simulink model "IARC_Nonlinear_Sensors"  (R2018a)
settings: Solver=ode1  StartTime=0.0  StopTime=20  FixedStep=T  RelTol=1e-3  EnableMultiTasking=on
undefined symbols (not defined in the file): A_1df, A_2df, alpha3, alpha_rp, alpha_x, alpha_z, an1, an1_v, an2, an3, bn1, bn1_v, bn2, bn3, dc_M_x, delta3, Epsilon3, F, g, Gamma1, Gamma2, Gamma3, Gamma4, gamma4_0, gamma_d_x, gamma_rp_0, gamma_x_0, gamma_z_0, Gammax, I, I_add, I_add_time, Jx, Jy, Jyaw, K, k1, k10, k11, k12, k2, k3, k4, k5, k6, k7, k8, k9, Ky, L, Light, LIMIT_CMD_PITCH, LIMIT_CMD_ROLL, LIMIT_CMD_xy, LIMIT_uCMD_HEIGHT, m, m_add, m_add_time, magnitude, MIL ... (+67)
libraries: simulink x131, simulink_extras x5, UAV_Control x4, aerolibwind2 x1
(part 6 of 6)

== system IARC_Nonlinear_Sensors/ARC Controller/Attitutde Control/pitch control/Adaptation Law_X/IARC, Physical Model Based Parameter Estimation (69)_pitch (theta)/Gamma/InitializationDelay ==
  u : Inport
  Clock : Clock
  Compare To Constant2 : simulink/Logic and Bit Operations/Compare To Constant  relop=>=  const=t0  OutDataTypeStr=boolean
  Data Type Conversion : DataTypeConversion
  Product : Product
  y : Outport
  wires:
  u/1 -> Product/1
  Compare To Constant2/1 -> Data Type Conversion/1
  Clock/1 -> Compare To Constant2/1
  Data Type Conversion/1 -> Product/2
  Product/1 -> y/1

== system IARC_Nonlinear_Sensors/ARC Controller/Attitutde Control/pitch control/Adaptation Law_X/IARC, Physical Model Based Parameter Estimation (69)_pitch (theta)/Gamma/vDv ==
  In1 : Inport
  Product2 : Product  Inputs=3  Multiplication=Matrix(*)
  Transpose2 : Math  Operator=transpose  SaturateOnIntegerOverflow=on
  eigenvector of Gamm_max : Constant  Value=v
  Out1 : Outport
  wires:
  Transpose2/1 -> Product2/1
  In1/1 -> Product2/2
  eigenvector of Gamm_max/1 -> Transpose2/1, Product2/3
  Product2/1 -> Out1/1

== system IARC_Nonlinear_Sensors/ARC Controller/Attitutde Control/roll control/Adaptation Law_Y/IARC, Physical Model Based Parameter Estimation (69)_roll (phi)/Gamma/Gamma_dot ==
  note: D.Gamma=mu1.G-mu2.G.P.P.G
      |
      | Normalized:
      | D.Gamma=alpha.G-(G.P.P.G)/(1+nu.P.GP)
  Phi_f : Inport
  Gamma : Inport  Port=2
  " " : Gain  Gain=mu2
  "  (Normalized)" : Gain  Gain=nu
  Add : Sum  Inputs=+-
  Add1 : Sum
  Add2 : Sum  Inputs=+-
  Constant : Constant
  Constant4 : Constant  Value=Norm_ON
  Divide : Product  Inputs=*/
  G.P.P.G : Product  Inputs=4  Multiplication=Matrix(*)
  Gamma1 : InportShadow  Port=2
  Gamma2 : InportShadow  Port=2
  P.G.P : Product  Inputs=3  Multiplication=Matrix(*)
  Switch2 : Switch  Threshold=0.5
  Transpose1 : Math  Operator=transpose  SaturateOnIntegerOverflow=on
  "forgetting factor " : Gain  Gain=mu1
  forgetting factor (Normalized) : Gain  Gain=alpha
  gamma_dot : Outport
  " 1+nu.Phi.G.Phi" : Outport  Port=2
  wires:
  "  (Normalized)"/1 -> Add1/2
  Phi_f/1 -> P.G.P/3, Transpose1/1, G.P.P.G/2
  Transpose1/1 -> P.G.P/1, G.P.P.G/3
  Gamma/1 -> G.P.P.G/1, P.G.P/2, G.P.P.G/4
  "forgetting factor "/1 -> Add/1
  G.P.P.G/1 -> " "/1, Divide/1
  Constant/1 -> Add1/1
  P.G.P/1 -> "  (Normalized)"/1
  Add1/1 -> Divide/2, " 1+nu.Phi.G.Phi"/1
  Gamma2/1 -> forgetting factor (Normalized)/1
  Add2/1 -> Switch2/1
  Constant4/1 -> Switch2/2
  Add/1 -> Switch2/3
  Switch2/1 -> gamma_dot/1
  Divide/1 -> Add2/2
  forgetting factor (Normalized)/1 -> Add2/1
  " "/1 -> Add/2
  Gamma1/1 -> "forgetting factor "/1

== system IARC_Nonlinear_Sensors/ARC Controller/Attitutde Control/roll control/Adaptation Law_Y/IARC, Physical Model Based Parameter Estimation (69)_roll (phi)/Gamma/InitializationDelay ==
  u : Inport
  Clock : Clock
  Compare To Constant2 : simulink/Logic and Bit Operations/Compare To Constant  relop=>=  const=t0  OutDataTypeStr=boolean
  Data Type Conversion : DataTypeConversion
  Product : Product
  y : Outport
  wires:
  u/1 -> Product/1
  Compare To Constant2/1 -> Data Type Conversion/1
  Clock/1 -> Compare To Constant2/1
  Data Type Conversion/1 -> Product/2
  Product/1 -> y/1

== system IARC_Nonlinear_Sensors/ARC Controller/Attitutde Control/roll control/Adaptation Law_Y/IARC, Physical Model Based Parameter Estimation (69)_roll (phi)/Gamma/vDv ==
  In1 : Inport
  Product2 : Product  Inputs=3  Multiplication=Matrix(*)
  Transpose2 : Math  Operator=transpose  SaturateOnIntegerOverflow=on
  eigenvector of Gamm_max : Constant  Value=v
  Out1 : Outport
  wires:
  Transpose2/1 -> Product2/1
  In1/1 -> Product2/2
  eigenvector of Gamm_max/1 -> Transpose2/1, Product2/3
  Product2/1 -> Out1/1

== system IARC_Nonlinear_Sensors/ARC Controller/Position Control/X control/Adaptation Law_X/IARC, Physical Model Based Parameter Estimation (69)_X/Gamma/Gamma_dot ==
  note: D.Gamma=mu1.G-mu2.G.P.P.G
      |
      | Normalized:
      | D.Gamma=alpha.G-(G.P.P.G)/(1+nu.P.GP)
  Phi_f : Inport
  Gamma : Inport  Port=2
  " " : Gain  Gain=mu2
  "  (Normalized)" : Gain  Gain=nu
  Add : Sum  Inputs=+-
  Add1 : Sum
  Add2 : Sum  Inputs=+-
  Constant : Constant
  Constant4 : Constant  Value=Norm_ON
  Divide : Product  Inputs=*/
  G.P.P.G : Product  Inputs=4  Multiplication=Matrix(*)
  Gamma1 : InportShadow  Port=2
  Gamma2 : InportShadow  Port=2
  P.G.P : Product  Inputs=3  Multiplication=Matrix(*)
  Switch2 : Switch  Threshold=0.5
  Transpose1 : Math  Operator=transpose  SaturateOnIntegerOverflow=on
  "forgetting factor " : Gain  Gain=mu1
  forgetting factor (Normalized) : Gain  Gain=alpha
  gamma_dot : Outport
  " 1+nu.Phi.G.Phi" : Outport  Port=2
  wires:
  "  (Normalized)"/1 -> Add1/2
  Phi_f/1 -> P.G.P/3, Transpose1/1, G.P.P.G/2
  Transpose1/1 -> P.G.P/1, G.P.P.G/3
  Gamma/1 -> G.P.P.G/1, P.G.P/2, G.P.P.G/4
  "forgetting factor "/1 -> Add/1
  G.P.P.G/1 -> " "/1, Divide/1
  Constant/1 -> Add1/1
  P.G.P/1 -> "  (Normalized)"/1
  Add1/1 -> Divide/2, " 1+nu.Phi.G.Phi"/1
  Gamma2/1 -> forgetting factor (Normalized)/1
  Add2/1 -> Switch2/1
  Constant4/1 -> Switch2/2
  Add/1 -> Switch2/3
  Switch2/1 -> gamma_dot/1
  Divide/1 -> Add2/2
  forgetting factor (Normalized)/1 -> Add2/1
  " "/1 -> Add/2
  Gamma1/1 -> "forgetting factor "/1

== system IARC_Nonlinear_Sensors/ARC Controller/Position Control/X control/Adaptation Law_X/IARC, Physical Model Based Parameter Estimation (69)_X/Gamma/InitializationDelay ==
  u : Inport
  Clock : Clock
  Compare To Constant2 : simulink/Logic and Bit Operations/Compare To Constant  relop=>=  const=t0  OutDataTypeStr=boolean
  Data Type Conversion : DataTypeConversion
  Product : Product
  y : Outport
  wires:
  u/1 -> Product/1
  Compare To Constant2/1 -> Data Type Conversion/1
  Clock/1 -> Compare To Constant2/1
  Data Type Conversion/1 -> Product/2
  Product/1 -> y/1

== system IARC_Nonlinear_Sensors/ARC Controller/Position Control/X control/Adaptation Law_X/IARC, Physical Model Based Parameter Estimation (69)_X/Gamma/vDv ==
  In1 : Inport
  Product2 : Product  Inputs=3  Multiplication=Matrix(*)
  Transpose2 : Math  Operator=transpose  SaturateOnIntegerOverflow=on
  eigenvector of Gamm_max : Constant  Value=v
  Out1 : Outport
  wires:
  Transpose2/1 -> Product2/1
  In1/1 -> Product2/2
  eigenvector of Gamm_max/1 -> Transpose2/1, Product2/3
  Product2/1 -> Out1/1

== system IARC_Nonlinear_Sensors/ARC Controller/Position Control/Y control/Adaptation Law_Y/IARC, Physical Model Based Parameter Estimation (69)_X/Gamma/Gamma_dot ==
  note: D.Gamma=mu1.G-mu2.G.P.P.G
      |
      | Normalized:
      | D.Gamma=alpha.G-(G.P.P.G)/(1+nu.P.GP)
  Phi_f : Inport
  Gamma : Inport  Port=2
  " " : Gain  Gain=mu2
  "  (Normalized)" : Gain  Gain=nu
  Add : Sum  Inputs=+-
  Add1 : Sum
  Add2 : Sum  Inputs=+-
  Constant : Constant
  Constant4 : Constant  Value=Norm_ON
  Divide : Product  Inputs=*/
  G.P.P.G : Product  Inputs=4  Multiplication=Matrix(*)
  Gamma1 : InportShadow  Port=2
  Gamma2 : InportShadow  Port=2
  P.G.P : Product  Inputs=3  Multiplication=Matrix(*)
  Switch2 : Switch  Threshold=0.5
  Transpose1 : Math  Operator=transpose  SaturateOnIntegerOverflow=on
  "forgetting factor " : Gain  Gain=mu1
  forgetting factor (Normalized) : Gain  Gain=alpha
  gamma_dot : Outport
  " 1+nu.Phi.G.Phi" : Outport  Port=2
  wires:
  "  (Normalized)"/1 -> Add1/2
  Phi_f/1 -> P.G.P/3, Transpose1/1, G.P.P.G/2
  Transpose1/1 -> P.G.P/1, G.P.P.G/3
  Gamma/1 -> G.P.P.G/1, P.G.P/2, G.P.P.G/4
  "forgetting factor "/1 -> Add/1
  G.P.P.G/1 -> " "/1, Divide/1
  Constant/1 -> Add1/1
  P.G.P/1 -> "  (Normalized)"/1
  Add1/1 -> Divide/2, " 1+nu.Phi.G.Phi"/1
  Gamma2/1 -> forgetting factor (Normalized)/1
  Add2/1 -> Switch2/1
  Constant4/1 -> Switch2/2
  Add/1 -> Switch2/3
  Switch2/1 -> gamma_dot/1
  Divide/1 -> Add2/2
  forgetting factor (Normalized)/1 -> Add2/1
  " "/1 -> Add/2
  Gamma1/1 -> "forgetting factor "/1

== system IARC_Nonlinear_Sensors/ARC Controller/Position Control/Y control/Adaptation Law_Y/IARC, Physical Model Based Parameter Estimation (69)_X/Gamma/InitializationDelay ==
  u : Inport
  Clock : Clock
  Compare To Constant2 : simulink/Logic and Bit Operations/Compare To Constant  relop=>=  const=t0  OutDataTypeStr=boolean
  Data Type Conversion : DataTypeConversion
  Product : Product
  y : Outport
  wires:
  u/1 -> Product/1
  Compare To Constant2/1 -> Data Type Conversion/1
  Clock/1 -> Compare To Constant2/1
  Data Type Conversion/1 -> Product/2
  Product/1 -> y/1

== system IARC_Nonlinear_Sensors/ARC Controller/Position Control/Y control/Adaptation Law_Y/IARC, Physical Model Based Parameter Estimation (69)_X/Gamma/vDv ==
  In1 : Inport
  Product2 : Product  Inputs=3  Multiplication=Matrix(*)
  Transpose2 : Math  Operator=transpose  SaturateOnIntegerOverflow=on
  eigenvector of Gamm_max : Constant  Value=v
  Out1 : Outport
  wires:
  Transpose2/1 -> Product2/1
  In1/1 -> Product2/2
  eigenvector of Gamm_max/1 -> Transpose2/1, Product2/3
  Product2/1 -> Out1/1

== system IARC_Nonlinear_Sensors/ARC Controller/Position Control/Z control/Estimate theta = K//m/IARC, Physical Model Based Parameter Estimation (69)/Gamma/Gamma_dot ==
  note: D.Gamma=mu1.G-mu2.G.P.P.G
      |
      | Normalized:
      | D.Gamma=alpha.G-(G.P.P.G)/(1+nu.P.GP)
  Phi_f : Inport
  Gamma : Inport  Port=2
  " " : Gain  Gain=mu2
  "  (Normalized)" : Gain  Gain=nu
  Add : Sum  Inputs=+-
  Add1 : Sum
  Add2 : Sum  Inputs=+-
  Constant : Constant
  Constant4 : Constant  Value=Norm_ON
  Divide : Product  Inputs=*/
  G.P.P.G : Product  Inputs=4  Multiplication=Matrix(*)
  Gamma1 : InportShadow  Port=2
  Gamma2 : InportShadow  Port=2
  P.G.P : Product  Inputs=3  Multiplication=Matrix(*)
  Switch2 : Switch  Threshold=0.5
  Transpose1 : Math  Operator=transpose  SaturateOnIntegerOverflow=on
  "forgetting factor " : Gain  Gain=mu1
  forgetting factor (Normalized) : Gain  Gain=alpha
  gamma_dot : Outport
  " 1+nu.Phi.G.Phi" : Outport  Port=2
  wires:
  "  (Normalized)"/1 -> Add1/2
  Phi_f/1 -> P.G.P/3, Transpose1/1, G.P.P.G/2
  Transpose1/1 -> P.G.P/1, G.P.P.G/3
  Gamma/1 -> G.P.P.G/1, P.G.P/2, G.P.P.G/4
  "forgetting factor "/1 -> Add/1
  G.P.P.G/1 -> " "/1, Divide/1
  Constant/1 -> Add1/1
  P.G.P/1 -> "  (Normalized)"/1
  Add1/1 -> Divide/2, " 1+nu.Phi.G.Phi"/1
  Gamma2/1 -> forgetting factor (Normalized)/1
  Add2/1 -> Switch2/1
  Constant4/1 -> Switch2/2
  Add/1 -> Switch2/3
  Switch2/1 -> gamma_dot/1
  Divide/1 -> Add2/2
  forgetting factor (Normalized)/1 -> Add2/1
  " "/1 -> Add/2
  Gamma1/1 -> "forgetting factor "/1

== system IARC_Nonlinear_Sensors/ARC Controller/Position Control/Z control/Estimate theta = K//m/IARC, Physical Model Based Parameter Estimation (69)/Gamma/InitializationDelay ==
  u : Inport
  Clock : Clock
  Compare To Constant2 : simulink/Logic and Bit Operations/Compare To Constant  relop=>=  const=t0  OutDataTypeStr=boolean
  Data Type Conversion : DataTypeConversion
  Product : Product
  y : Outport
  wires:
  u/1 -> Product/1
  Compare To Constant2/1 -> Data Type Conversion/1
  Clock/1 -> Compare To Constant2/1
  Data Type Conversion/1 -> Product/2
  Product/1 -> y/1

== system IARC_Nonlinear_Sensors/ARC Controller/Position Control/Z control/Estimate theta = K//m/IARC, Physical Model Based Parameter Estimation (69)/Gamma/vDv ==
  In1 : Inport
  Product2 : Product  Inputs=3  Multiplication=Matrix(*)
  Transpose2 : Math  Operator=transpose  SaturateOnIntegerOverflow=on
  eigenvector of Gamm_max : Constant  Value=v
  Out1 : Outport
  wires:
  Transpose2/1 -> Product2/1
  In1/1 -> Product2/2
  eigenvector of Gamm_max/1 -> Transpose2/1, Product2/3
  Product2/1 -> Out1/1

== matlab function IARC_Nonlinear_Sensors/Sensors and Filters/Data processing/Estimate Position/Extrapolation - x ==
  settings: updateMethod=DISCRETE
  data: xin input; xout output; xdotin input; dt input; new input; isTracking input
function xout = fcn(xin, xdotin, dt, new, isTracking)
%#codegen

%
% Pass through input if "new" data available and OptiTrack is tracking.
% Otherwise, use linear interpolation to estimate the signal value and
% ignore the input data.
%
persistent x;

if( isempty(x) )
    x = 0;
end;

if( new == 1 && isTracking == 1 )
    x = xin;
else
    x = x+dt*xdotin;
end;

xout = x;

== matlab function IARC_Nonlinear_Sensors/Sensors and Filters/Data processing/Estimate Position/Extrapolation - z ==
  settings: updateMethod=DISCRETE  sampleTime=T
  data: xin input; xout output; xdotin input; dt input; new input; isTracking input
function xout = fcn(xin, xdotin, dt, new, isTracking)
%#codegen

%
% Pass through input if "new" data available and OptiTrack is tracking.
% Otherwise, use linear interpolation to estimate the signal value and
% ignore the input data.
%
persistent x;

if( isempty(x) )
    x = 0;
end;

if( new == 1 && isTracking == 1 )
    x = xin;
else
    x = x+dt*xdotin;
end;

xout = x;

== matlab function IARC_Nonlinear_Sensors/Sensors and Filters/Data processing/Estimate Attitude/Kalman Filter - Pitch ==
  settings: updateMethod=DISCRETE  sampleTime=T
  data: angle output; acc_angle input; gyro_rate input; opti_angle input; Euler input; dt input
function angle   = fcn(acc_angle,gyro_rate,opti_angle,Euler,dt)
%#eml
    % a bias in the accelerometer will result in a bias in the filter
    % estimate
    Q_angle = 0.01;
    Q_gyro   = 0.01; %0.01;  %0.003
    R_angle  =  0.001;  %0.03

    
    persistent P_00;
    persistent P_01;
    persistent P_10;
    persistent P_11;
    persistent x_angle;
    persistent x_bias;
        
    if isempty(P_00)
        P_00 = 0;
    end
    
    if isempty(P_01)
        P_01 = 0;
    end
    if isempty(P_10)
        P_10 = 0;
    end
    if isempty(P_11)
        P_11 = 0;
    end
     if isempty(x_bias)
        x_bias = 0;
     end
     if isempty(x_angle)
        x_angle = 0;
     end
    
    
    % Calculate the new output
    x_angle = x_angle + dt * (-gyro_rate(1)*sin(Euler(2))*tan(Euler(1))+gyro_rate(2)+gyro_rate(3)*cos(Euler(2))*tan(Euler(1)) - x_bias);%
    P_00 = P_00 -  dt * (P_10 + P_01) + Q_angle * dt;
    P_01 = P_01  - dt * P_11;
    P_10 = P_10  - dt * P_11;
    P_11 = P_11  + Q_gyro * dt;

    % Assuming H = [0.98 (effect of gyro) 0.02 (effect of acc)]
    %e = (0.97*x_angle + 0.03*acc_angle) - x_angle;
    e = (0.9*x_angle + 0.01*acc_angle + 0.09*opti_angle) - x_angle;
    S = P_00 + R_angle;
    K_0 = P_00 / S;
    K_1 = P_10 / S;

    % Correction
    x_angle = x_angle+  K_0 * e;
    x_bias  = x_bias+  K_1 * e;
    P_00 = P_00 - K_0 * P_00;
    P_01 = P_01 - K_0 * P_01;
    P_10 = P_10 - K_1 * P_00;
    P_11 = P_11 - K_1 * P_01;

    angle = x_angle;

== matlab function IARC_Nonlinear_Sensors/Sensors and Filters/Data processing/Estimate Position/Extrapolation - y ==
  settings: updateMethod=DISCRETE  sampleTime=T
  data: xin input; xout output; xdotin input; dt input; new input; isTracking input
function xout = fcn(xin, xdotin, dt, new, isTracking)
%#codegen

%
% Pass through input if "new" data available and OptiTrack is tracking.
% Otherwise, use linear interpolation to estimate the signal value and
% ignore the input data.
%
persistent x;

if( isempty(x) )
    x = 0;
end;

if( new == 1 && isTracking == 1 )
    x = xin;
else
    x = x+dt*xdotin;
end;

xout = x;

== matlab function IARC_Nonlinear_Sensors/Sensors and Filters/Data processing/Estimate Attitude/Kalman Filter - Roll ==
  settings: updateMethod=DISCRETE  sampleTime=T
  data: angle output; acc_angle input; gyro_rate input; opti_angle input; Euler input; dt input
function angle    = fcn(acc_angle,gyro_rate,opti_angle,Euler,dt)
%#eml

    Q_angle = 0.01;
    Q_gyro   = 0.01; %0.01;  %0.003
    R_angle  =  0.001;  %0.03

    
    persistent P_00;
    persistent P_01;
    persistent P_10;
    persistent P_11;
    persistent x_angle;
    persistent x_bias;
        
    if isempty(P_00)
        P_00 = 8*10^-4*0;
    end
    
    if isempty(P_01)
        P_01 = -8*10^-4*0;
    end
    if isempty(P_10)
        P_10 = -8*10^-4*0;
    end
    if isempty(P_11)
        P_11 = 0.01*0;
    end
     if isempty(x_bias)
        x_bias = 0;
     end
     if isempty(x_angle)
        x_angle = 0;
     end
    
    
    % Calculate the new output
    x_angle = x_angle + dt * (gyro_rate(1)*cos(Euler(2))-gyro_rate(3)*sin(Euler(2)) - x_bias);
    P_00 = P_00 -  dt * (P_10 + P_01) + Q_angle * dt;
    P_01 = P_01  - dt * P_11;
    P_10 = P_10  - dt * P_11;
    P_11 = P_11  + Q_gyro * dt;

    % Assuming H = [0.97 (effect of gyro) 0.03 (effect of acc)]
    %e = (0.97*x_angle + 0.03*acc_angle) - x_angle;
    e = (0.9*x_angle + 0.01*acc_angle + 0.09*opti_angle) - x_angle;
    S = P_00 + R_angle;
    K_0 = P_00 / S;
    K_1 = P_10 / S;

    % Correction
    x_angle = x_angle+  K_0 * e;
    x_bias  = x_bias+  K_1 * e;
    P_00 = P_00 - K_0 * P_00;
    P_01 = P_01 - K_0 * P_01;
    P_10 = P_10 - K_1 * P_00;
    P_11 = P_11 - K_1 * P_01;

    angle = x_angle;
    P=[P_00 P_01;P_10 P_11];

== matlab function IARC_Nonlinear_Sensors/Sensors and Filters/Data processing/Estimate Attitude/Kalman Filter - Yaw ==
  settings: updateMethod=DISCRETE  sampleTime=T
  data: angle output; opti_angle input; gyro_rate input; Euler input; dt input
function angle   = fcn(opti_angle,gyro_rate,Euler,dt)
%#eml

     Q_angle  = 0.01; %0.01; %0.001
     Q_gyro   = 0.01; %0.01;  %0.003
     R_angle  =  0.001;  %0.03

    
    persistent P_00;
    persistent P_01;
    persistent P_10;
    persistent P_11;
    persistent x_angle;
    persistent x_bias;
        
    if isempty(P_00)
        P_00 = 0;
    end
    
    if isempty(P_01)
        P_01 = 0;
    end
    if isempty(P_10)
        P_10 = 0;
    end
    if isempty(P_11)
        P_11 = 0;
    end
     if isempty(x_bias)
        x_bias = 0;
     end
     if isempty(x_angle)
        x_angle = 0;
     end
    
    
    % Calculate the new output
    x_angle = x_angle + dt * ( gyro_rate(1)*sin(Euler(2))/cos(Euler(1))+gyro_rate(3)*cos(Euler(2))/cos(Euler(1)) - x_bias); % 
    P_00 = P_00 -  dt * (P_10 + P_01) + Q_angle * dt;
    P_01 = P_01  - dt * P_11;
    P_10 = P_10  - dt * P_11;
    P_11 = P_11  + Q_gyro * dt;

    % Assuming H = [0.98 (effect of gyro) 0.02 (effect of acc)]
    e = (0.99*x_angle + 0.01*opti_angle) - x_angle;
    S = P_00 + R_angle;
    K_0 = P_00 / S;
    K_1 = P_10 / S;

    % Correction
    x_angle = x_angle+  K_0 * e;
    x_bias  = x_bias+  K_1 * e;
    P_00 = P_00 - K_0 * P_00;
    P_01 = P_01 - K_0 * P_01;
    P_10 = P_10 - K_1 * P_00;
    P_11 = P_11 - K_1 * P_01;

    angle = x_angle;

== matlab function IARC_Nonlinear_Sensors/Sensors and Filters/Data processing/Estimate Attitude/Calculate Roll and Pitch (From Acceleration Data)/calc_roll_pitch ==
  data: roll_acc output; pitch_acc output; acc_body input
function [roll_acc, pitch_acc]   = fcn(acc_body)
%#eml
n = norm(acc_body,2);
if n>eps
    acc_body = -acc_body/n; 
else
    acc_body = [0 0 1]';
end

roll_acc = atan2(acc_body(2),acc_body(3));
pitch_acc = atan2( -acc_body(1), acc_body(2)*sin(roll_acc)+acc_body(3)*cos(roll_acc));

== matlab function IARC_Nonlinear_Sensors/Sensors and Filters/Data processing/Estimate Position/Kalman Filter - Height ==
  settings: updateMethod=DISCRETE  sampleTime=T
  data: height output; optitrack input; sonar_d input; dt input
function height   = fcn(optitrack,sonar_d,dt)
%#eml

     Q_sonar  = 0.1; %0.01; %0.001
     Q_optitrack   = 0.01; %0.01;  %0.003
     R_height =  0.03;  %0.03

    
    persistent P_00;
    persistent P_01;
    persistent P_10;
    persistent P_11;
    persistent x_height;
    persistent x_bias;
        
    if isempty(P_00)
        P_00 = 0;
    end
    
    if isempty(P_01)
        P_01 = 0;
    end
    if isempty(P_10)
        P_10 = 0;
    end
    if isempty(P_11)
        P_11 = 0;
    end
    if isempty(x_bias)
       x_bias = 0;
    end
    if isempty(x_height)
       x_height = 0;
    end
    
    
    % Compensate for sonar rate calculation (sonar sample rate is 10Hz)
    sonar_d_corrected = sonar_d*dt*10;  % m/s
    
    % Reject large height rate changes from sonar
    % As those are likely a result of obstacle underneath or noise
    if(abs(sonar_d_corrected) > 1 )    % max height rate (m/s)
        sonar_d_corrected = 0;
    end
    
    % Calculate the new output
    %x_height = x_height + dt * (sonar_d - x_bias); % old 
    x_height = x_height + dt * (sonar_d_corrected - x_bias);
    P_00 = P_00 -  dt * (P_10 + P_01) + Q_sonar * dt;
    P_01 = P_01  - dt * P_11;
    P_10 = P_10  - dt * P_11;
    P_11 = P_11  + Q_optitrack * dt;

    % Assuming H = [0.95 (effect of optitrack) 0.05 (effect of sonar)]
    e = (0.05*x_height + 0.95*optitrack) - x_height;
    S = P_00 + R_height;
    K_0 = P_00 / S;
    K_1 = P_10 / S;

    % Correction
    x_height = x_height+  K_0 * e;
    x_bias  = x_bias+  K_1 * e;
    P_00 = P_00 - K_0 * P_00;
    P_01 = P_01 - K_0 * P_01;
    P_10 = P_10 - K_1 * P_00;
    P_11 = P_11 - K_1 * P_01;

    height = x_height;

== matlab function IARC_Nonlinear_Sensors/Sensors and Filters/Data processing/Estimate Attitude/Calculate Roll and Pitch (From Acceleration Data)/calc_roll_pitch_asin ==
  data: roll_acc output; pitch_acc output; acc_body input
function [roll_acc, pitch_acc]   = fcn(acc_body)
%#eml

roll_acc = asin(-acc_body(2)/9.8);

pitch_acc = asin(acc_body(1)/9.8);
